simulink model "IO503hybrid"  (R2012b)
settings: Solver=FixedStepDiscrete  StartTime=0.0  StopTime=inf  RelTol=1e-3
InitFcn:
  | Ts = 0.1;
undefined symbols (not defined in the file): standard
libraries: speedgoatlib x10, xpcseriallib x4, simulink x2, xpclib x2
settings Model: BufferReuse=off  Creator=dkuratli  LastModifiedBy=lab3
settings SolverCC: EnableConcurrentExecution=on
settings OptimizationCC: BlockReduction=off  OptimizeBlockIOStorage=off  BufferReuse=off  ExpressionFolding=off  ExpressionDepthLimit=128  LocalBlockOutputs=off
settings DebuggingCC: StateNameClashWarn=none
settings HardwareCC: ProdIntDivRoundTo=Zero  ProdEndianess=LittleEndian  ProdHWDeviceType=Generic->32-bit x86 compatible
settings RTWCC: SystemTargetFile=xpctarget.tlc  TemplateMakefile=xpc_default_tmf  Description=Simulink Real-Time  RTWVerbose=off  ProcessScript=xpctarget_make_rtw_hook  RTWCompilerOptimization=On
settings CodeAppCC: CustomSymbolStrType=$N$R$M_T
settings xpcTargetCC: TargetFcnLib=ansi_tfl_table_tmw.mat  CodeReplacementLibrary=XPC_BLAS  ParMdlRefBuildCompliant=on  ConcurrentExecutionCompliant=on  CombineSignalStateStructs=off  GRTInterface=on  GenerateAllocFcn=off  xPCTaskExecutionProfile=off  xPCRL32EventNumber=5000  xPCLoadParamSetFile=off  xPCConcurrentTasks=off  xPCEnableSFAnimation=off

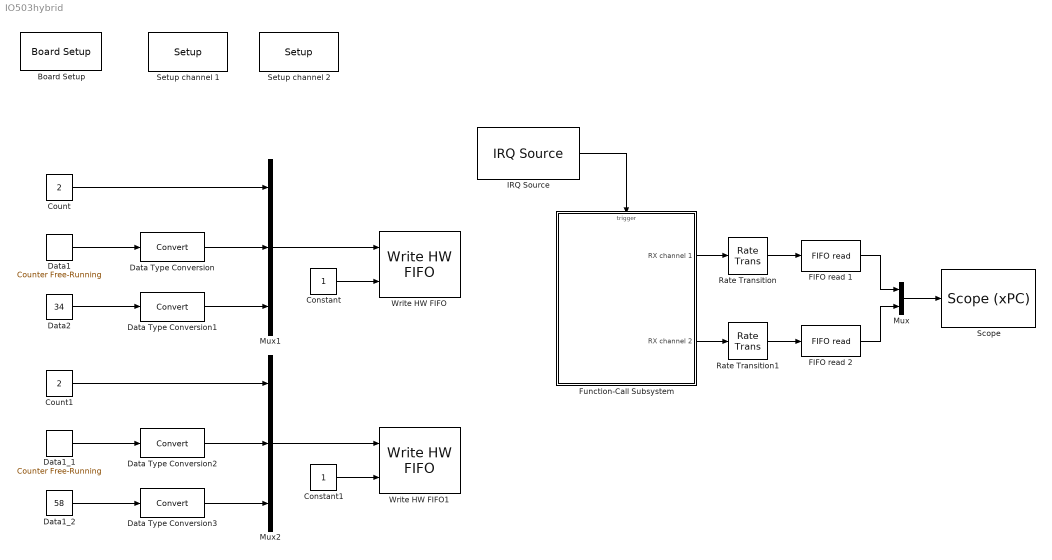
== system IO503hybrid ==
  Board Setup : speedgoatlib/IO503/Speedgoat IO503 Internal blocks/Board Setup  irqnum=10  slot=-1
  Constant : Constant  OutDataTypeStr=Inherit: Inherit via back propagation  SampleTime=Ts
  Constant1 : Constant  OutDataTypeStr=Inherit: Inherit via back propagation  SampleTime=Ts
  Count : Constant  Value=2  OutDataTypeStr=Inherit: Inherit via back propagation  SampleTime=Ts
  Count1 : Constant  Value=2  OutDataTypeStr=Inherit: Inherit via back propagation  SampleTime=Ts
  Data Type Conversion{,1..3} (4 alike) : DataTypeConversion
  Data1 : simulink/Sources/Counter Free-Running  NumBits=8  tsamp=Ts
  Data1_1 : simulink/Sources/Counter Free-Running  NumBits=8  tsamp=Ts
  Data1_2 : Constant  Value=58  OutDataTypeStr=Inherit: Inherit via back propagation  SampleTime=Ts
  Data2 : Constant  Value=34  OutDataTypeStr=Inherit: Inherit via back propagation  SampleTime=Ts
  FIFO read 1 : xpcseriallib/FIFO read   maxsize=2  minsize=1  usedelimiter=off  delimiter=13  outputtype=count+32 bit int  enable=off  enableout=off  sampletime=-1
  FIFO read 2 : xpcseriallib/FIFO read   maxsize=2  minsize=1  usedelimiter=off  delimiter=13  outputtype=count+32 bit int  enable=off  enableout=off  sampletime=-1
  Function-Call Subsystem : Subsystem  TreatAsAtomicUnit=on
  IRQ Source : xpclib/Asynchronous Event/IRQ Source  irqNo=10  preempt=10  b_type=None/Other  slot=-1
  Mux : Mux  Inputs=2
  Mux1 : Mux  Inputs=3
  Mux2 : Mux  Inputs=3
  Rate Transition : RateTransition  Integrity=off  Deterministic=off  OutPortSampleTime=0
  Rate Transition1 : RateTransition  Integrity=off  Deterministic=off  OutPortSampleTime=0
  "Scope " : xpclib/Misc./Scope (xPC)   scopeno=1  scopetype=Target  autostart=on  viewmode=Numerical  formatstr='%15.6f'  grid=on  ylimits=[0,0]  nosamples=3  noprepostsamples=0  interleave=1  triggermode=FreeRun  triggersignal=1  trigsignalfromport=off  triggerlevel=0.0  triggerslope=Either  triggerscope=1  triggersample=0  filename=data.dat  mode=Lazy  writesize=512  autorestart=off  dynamicfilemode=off  maxwritefilesize=512*1024^2
  "Setup channel 1 " : speedgoatlib/IO503/Speedgoat IO503 Internal blocks/Setup  port=1  transceiver=RS232 (max 921.6kb/s)  standard=on  baudrate=921600  bauddivisor=1  mode8x=16x (standard)  prescale=off  width=8  nstop=1  parity=None  rlevel=1  ctsmode=none  xonoff=none  xon=17  xoff=19  rs485mode=off  rs485delay=0  slot=-1
  Setup channel 2 : speedgoatlib/IO503/Speedgoat IO503 Internal blocks/Setup  port=2  transceiver=RS232 (max 921.6kb/s)  standard=on  baudrate=921600  bauddivisor=1  mode8x=16x (standard)  prescale=off  width=8  nstop=1  parity=None  rlevel=1  ctsmode=none  xonoff=none  xon=17  xoff=19  rs485mode=off  rs485delay=0  slot=-1
  Write HW FIFO : speedgoatlib/IO503/Speedgoat IO503 Internal blocks/Write HW FIFO  port=1  slot=-1
  Write HW FIFO1 : speedgoatlib/IO503/Speedgoat IO503 Internal blocks/Write HW FIFO  port=2  slot=-1
  wires:
  IRQ Source/1 -> Function-Call Subsystem/Trigger
  Constant/1 -> Write HW FIFO/2
  Mux1/1 -> Write HW FIFO/1
  Count/1 -> Mux1/1
  Data2/1 -> Data Type Conversion1/1
  Data Type Conversion/1 -> Mux1/2
  Data Type Conversion1/1 -> Mux1/3
  Rate Transition/1 -> FIFO read 1/1
  Data1/1 -> Data Type Conversion/1
  Rate Transition1/1 -> FIFO read 2/1
  Function-Call Subsystem/1(RX channel 1) -> Rate Transition/1
  Function-Call Subsystem/2(RX channel 2) -> Rate Transition1/1
  Constant1/1 -> Write HW FIFO1/2
  Mux2/1 -> Write HW FIFO1/1
  Count1/1 -> Mux2/1
  Data1_2/1 -> Data Type Conversion3/1
  Data Type Conversion2/1 -> Mux2/2
  Data Type Conversion3/1 -> Mux2/3
  Data1_1/1 -> Data Type Conversion2/1
  FIFO read 1/1 -> Mux/1
  FIFO read 2/1 -> Mux/2
  Mux/1 -> "Scope "/1

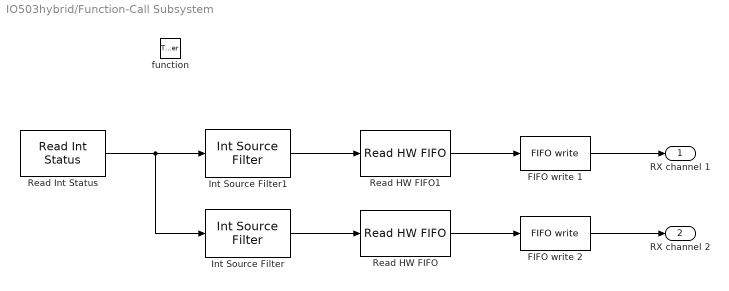
== system IO503hybrid/Function-Call Subsystem ==
  function : TriggerPort  TriggerType=function-call
  FIFO write 1 : xpcseriallib/FIFO write   size=64  inputtype=count+32 bit uint  present=off  sampletime=-1  id=RCV channel 2
  FIFO write 2 : xpcseriallib/FIFO write   size=64  inputtype=count+32 bit uint  present=off  sampletime=-1  id=RCV channel 2
  Int Source Filter : speedgoatlib/IO503/Speedgoat IO503 Internal blocks/Int Source Filter  port=2  value=Receive data
  Int Source Filter1 : speedgoatlib/IO503/Speedgoat IO503 Internal blocks/Int Source Filter  port=1  value=Receive data
  Read HW FIFO : speedgoatlib/IO503/Speedgoat IO503 Internal blocks/Read HW FIFO  port=2  flush=on  slot=-1
  Read HW FIFO1 : speedgoatlib/IO503/Speedgoat IO503 Internal blocks/Read HW FIFO  port=1  flush=on  slot=-1
  Read Int Status : speedgoatlib/IO503/Speedgoat IO503 Internal blocks/Read Int Status  slot=-1
  RX channel 1 : Outport
  RX channel 2 : Outport  Port=2
  wires:
  Read Int Status/1 -> Int Source Filter/1, Int Source Filter1/1
  Int Source Filter/1 -> Read HW FIFO/1
  Read HW FIFO/1 -> FIFO write 2/1
  FIFO write 2/1 -> RX channel 2/1
  Int Source Filter1/1 -> Read HW FIFO1/1
  Read HW FIFO1/1 -> FIFO write 1/1
  FIFO write 1/1 -> RX channel 1/1
